simulink model "mqsls_sim_actual"  (R2024b)
settings: configuration reference "prj_default_config" (kept outside this file)
settings Model: Creator=yangyu  LastModifiedBy=yangyu
settings ConfigSetRef: SourceName=prj_default_config  SourceLocation=Base Workspace

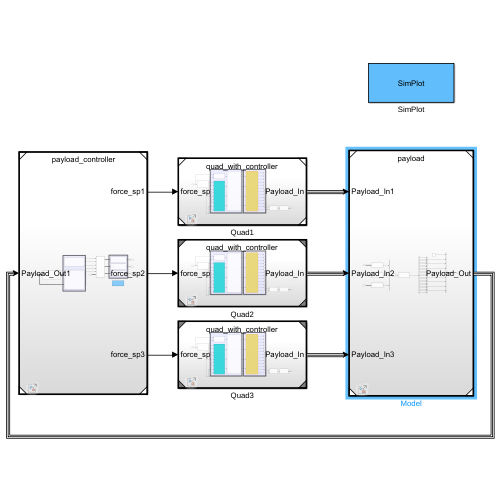
[thumbnail: Simulink's stored preview of the top-level diagram]
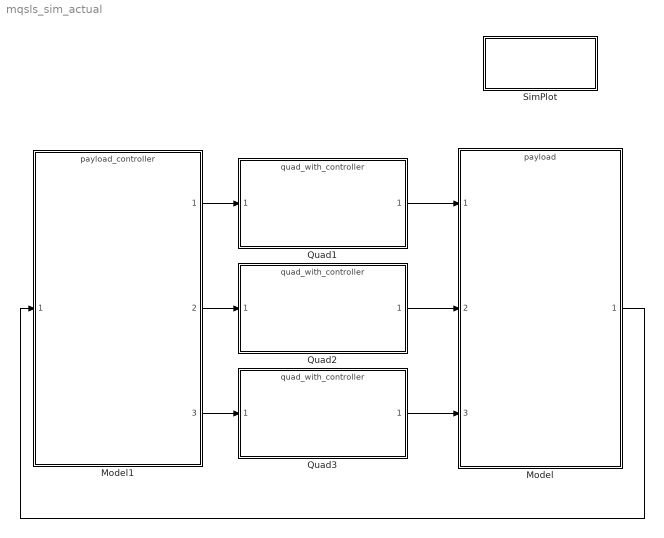
== system mqsls_sim_actual ==
  Model : ModelReference  ModelNameDialog=payload.slx  SimulationMode=Normal  ModelReferenceVersion=1.90
  Model1 : ModelReference  ModelNameDialog=payload_controller.slx  SimulationMode=Normal  ModelReferenceVersion=1.266
  Quad1 : ModelReference  ModelNameDialog=quad_with_controller  SimulationMode=Normal  ModelReferenceVersion=1.84
  Quad2 : ModelReference  ModelNameDialog=quad_with_controller  SimulationMode=Normal  ModelReferenceVersion=1.84
  Quad3 : ModelReference  ModelNameDialog=quad_with_controller  SimulationMode=Normal  ModelReferenceVersion=1.84
  SimPlot : Subsystem
      settings: OpenFcn=run('simplot.m');
      mask Display: disp('SimPlot');
  wires:
  Quad1/1 -> Model/1
  Model1/1 -> Quad1/1
  Quad2/1 -> Model/2
  Model1/2 -> Quad2/1
  Quad3/1 -> Model/3
  Model1/3 -> Quad3/1
  Model/1 -> Model1/1

== system mqsls_sim_actual/SimPlot ==
